simulink model "flowheater_demo"  (R2016a)
settings: Solver=VariableStepAuto  StartTime=0.0  StopTime=43680  MaxStep=1  MinStep=0.1  RelTol=1e-3
PreLoadFcn:
  | global N P0d P0L Pout P1 d
  | load flowheater_demo.mat
values from neighbouring files (symbols this model uses):
  Teg = [502.945679 502.511047 502.24646 502.038605 502.095306 502.548828 503.059082 503.266968 502.889008 502.492157 502.189789 502.133087 ... (1458 elements, 729x2)]    [flowheater_demo.mat]
  Tw = [53.106552 53.020687 52.913349 52.827469 52.827469 52.881145 52.945553 53.020687 53.042164 53.031414 53.042164 52.988483 ... (1458 elements, 729x2)]    [flowheater_demo.mat]
libraries: simulink x4
settings Model: Creator=ivand  LastModifiedBy=ivand

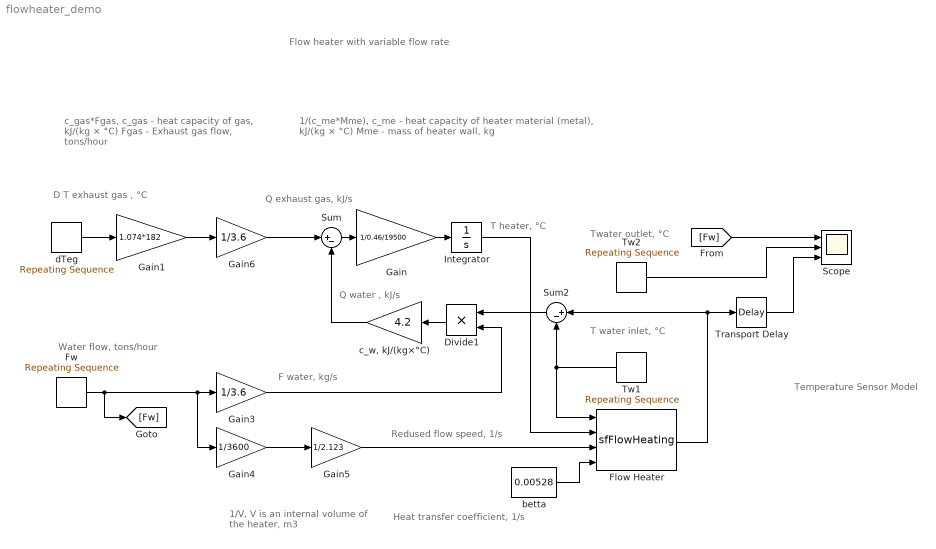
== system flowheater_demo ==
  note: Flow heater with variable flow rate
  note: c_gas*Fgas,
      | c_gas - heat capacity of gas, kJ/(kg × °С)
      | Fgas - Exhaust gas flow, tons/hour
  note: 1/V,  V is an internal
      | volume of the heater, m3
  note: Temperature
      | Sensor Model
  note: D T exhaust
      | gas , °С
  note: Heat transfer
      | coefficient, 1/s
  note: Water flow,
      | tons/hour
  note: Q water ,
      | kJ/s
  note: Redused flow speed, 1/s
  note: T heater, °С
  note: Q exhaust
      | gas, kJ/s
  note: F water, kg/s
  note: Twater outlet, °С
  note: T water inlet, °С
  note: 1/(c_me*Mme),
      | c_me - heat capacity of heater material (metal), kJ/(kg × °С)
      | Mme - mass of heater wall, kg
  Divide1 : Product  Inputs=**
  Flow Heater : M-S-Function  FunctionName=sfFlowHeating
  Fw : simulink/Sources/Repeating Sequence  rep_seq_t=t  rep_seq_y=Fw
  Gain : Gain  Gain=1/0.46/19500
  Gain1 : Gain  Gain=1.074*182
  Gain3 : Gain  Gain=1/3.6
  Gain4 : Gain  Gain=1/3600
  Gain5 : Gain  Gain=1/2.123
  Gain6 : Gain  Gain=1/3.6
  Integrator : Integrator  InitialCondition=Tw(1,2)
  Scope : Scope  NumInputPorts=3
  Sum : Sum  Inputs=|+-
  Sum2 : Sum  Inputs=|+-
  Transport Delay : TransportDelay  DelayTime=90
  Tw1 : simulink/Sources/Repeating Sequence  rep_seq_t=t  rep_seq_y=Tw(:,1)
  Tw2 : simulink/Sources/Repeating Sequence  rep_seq_t=t  rep_seq_y=Tw(:,2)
  betta : Constant  Value=0.00528
  "c_w, kJ/(kg×°С)" : Gain  Gain=4.2
  dTeg : simulink/Sources/Repeating Sequence  rep_seq_t=t  rep_seq_y=Teg(:,1)-Teg(:,2)
  wires:
  betta/1 -> Flow Heater/4
  Tw1/1 -> Sum2/2, Flow Heater/1
  Fw/1 -> [Fw], Gain4/1, Gain3/1
  Integrator/1 -> Flow Heater/2
  Gain/1 -> Integrator/1
  Sum/1 -> Gain/1
  dTeg/1 -> Gain1/1
  "c_w, kJ/(kg×°С)"/1 -> Sum/2
  Divide1/1 -> "c_w, kJ/(kg×°С)"/1
  Gain3/1 -> Divide1/2
  Gain5/1 -> Flow Heater/3
  Sum2/1 -> Divide1/1
  Flow Heater/1 -> Sum2/1, Transport Delay/1
  Gain4/1 -> Gain5/1
  Transport Delay/1 -> Scope/3
  Gain1/1 -> Gain6/1
  Gain6/1 -> Sum/1
  Tw2/1 -> Scope/2
  [Fw] -> Scope/1
